simulink model "cf_main_7_2"  (R2022a)
settings: Solver=FixedStepAuto  StartTime=0.0  StopTime=simTime  FixedStep=sample_time  RelTol=1e-3
model workspace: external: MAT-File (data not in the file)
undefined symbols (not defined in the file or in its folder): Angular, g, l0, l1, Linear, mass_total, poly_traj, pos_Kd, pos_Ki, pos_Kp, pos_Kvel, pos_N, pos_sat, Pose, Position, posx_Kd, posx_Ki, posx_Kp, posy_Kd, posy_Ki, posy_Kp, posz_Kd, posz_Ki, posz_Kp, publish_rate, quat2rotm, simTime
libraries: robotlib x11, slpidlib x4, simulink_extras x3, simulink x1, vrlib x1
settings Model: Creator=david  LastModifiedBy=dtu31390
settings SolverCC: AlgebraicLoopSolver=TrustRegion
settings DataIOCC: LimitDataPoints=on  MaxDataPoints=10000
settings OptimizationCC: EnhancedBackFolding=on  PassReuseOutputArgsThreshold=0  ZeroExternalMemoryAtStartup=off  ZeroInternalMemoryAtStartup=off  MaxStackSize=64  OptimizeBlockOrder=speed  DifferentSizesBufferReuse=on
settings DebuggingCC: ParameterTunabilityLossMsg=error  UnconnectedInputMsg=warning  UnconnectedOutputMsg=warning  UnconnectedLineMsg=warning  AllowSymbolicDim=off  SFUnexpectedBacktrackingDiag=warning  SFNoUnconditionalDefaultTransitionDiag=warning  SFExecutionAtInitializationDiag=none  SFMachineParentedDataDiag=warning  UnderSpecifiedDimensionMsg=warning  ArithmeticOperatorsInVariantConditions=warning
settings HardwareCC: ProdBitPerPointer=32  ProdBitPerSizeT=32  ProdBitPerPtrDiffT=32  ProdLargestAtomicFloat=None  ProdIntDivRoundTo=Undefined  ProdEndianess=Unspecified  ProdWordSize=32  ProdHWDeviceType=Generic->Unspecified (assume 32-bit Generic)  UseEmbeddedCoderFeatures=off
settings SFSimCC: SimUseLocalCustomCode=off  MATLABDynamicMemAlloc=off  CustomCodeUndefinedFunction=UseInterfaceOnly  SimTargetLang=C++
settings RTWCC: SystemTargetFile=ert.tlc  HardwareBoard=Robot Operating System (ROS)  TLCOptions="-aInlineSetEventsForThisBaseRateFcn=TLC_FALSE -aSuppressMultiTaskScheduler=TLC_FALSE  -aRateBasedStepFcn=0"  TemplateMakefile=ert_default_tmf  RTWUseLocalCustomCode=off  Toolchain=Catkin  TargetLang=C++  DLArmComputeVersion=19.05
settings CodeAppCC: ForceParamTrailComments=on  OperatorAnnotations=on
settings ERTTargetCC: ERTCustomFileBanners=off  CodeInterfacePackaging=C++ class  SupportContinuousTime=on  SupportNonInlinedSFcns=on  RemoveResetFunc=off  ModelStepFunctionPrototypeControlCompliant=off  RootIOFormat=Structure reference
settings ConfigComp: CovMetricSettings=dw  CovSaveCumulativeToWorkspaceVar=on  CovSaveSingleToWorkspaceVar=on  CovExternalEMLEnable=off  CovSFcnEnable=off
settings SimscapeCC: SimscapeLogType=all  SimscapeLogSimulationStatistics=on  SimscapeLogDataHistory=10000
settings ExplorerConfigSet: InternalSimMechanicsExplorerSettings="<ExplorerConfiguration><canonicalview>default</canonicalview><AnimationSetting><BasePlaybackSpeed>1.0</BasePlaybackSpeed><PlaybackSpeedFactor>1.0</PlaybackSpeedFactor></AnimationSetting><TilePanel><TileInfo><Tiles Columns=\"1\" Count=\"1\" Rows=\"1\"><Column Weight=\"1\"/><Row Weight=\"1\"/><Tile Height=\"1\" Width=\"1\" X=\"0\" Y=\"0\"/></Tiles></TileInfo><SceneInfo><SceneViewer><BGColor><R>0.400000005960464478</R><G>0.400000005960464478</G><B>0.400000005960464478</B></BGColor><Camera><DoPerspective>off</DoPerspective><Position><X>7.41918867546502359</X><Y>0.562842449888731333</Y><Z>8.36768126399918444</Z></Position><Center><X>4.24878770726833288</X><Y>4.27540210027623324</Y><Z>0.996100590645515815</Z></Center><Up><X>-0.578313069199200891</X><Y>0.601173295476169489</Y><Z>0.551493121262380703</Z></Up><ViewLimDist>1</ViewLimDist><YLim>5.48746925830841104</YLim><XLim>8.41878250057976274</XLim></Camera></SceneViewer></SceneInfo></TilePanel><MechEditorPanel><Cameras/><GfxPanelCameraMap/><VideoCreator><PlaybackSpeedRatio>1.0</PlaybackSpeedRatio><FrameRate>30</FrameRate><VideoFormat>Motion JPEG AVI</VideoFormat><FrameSize>auto</FrameSize></VideoCreator></MechEditorPanel></ExplorerConfiguration>"

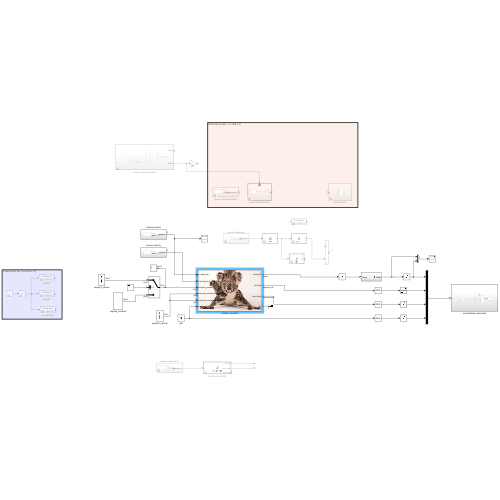
[thumbnail: Simulink's stored preview of the top-level diagram]
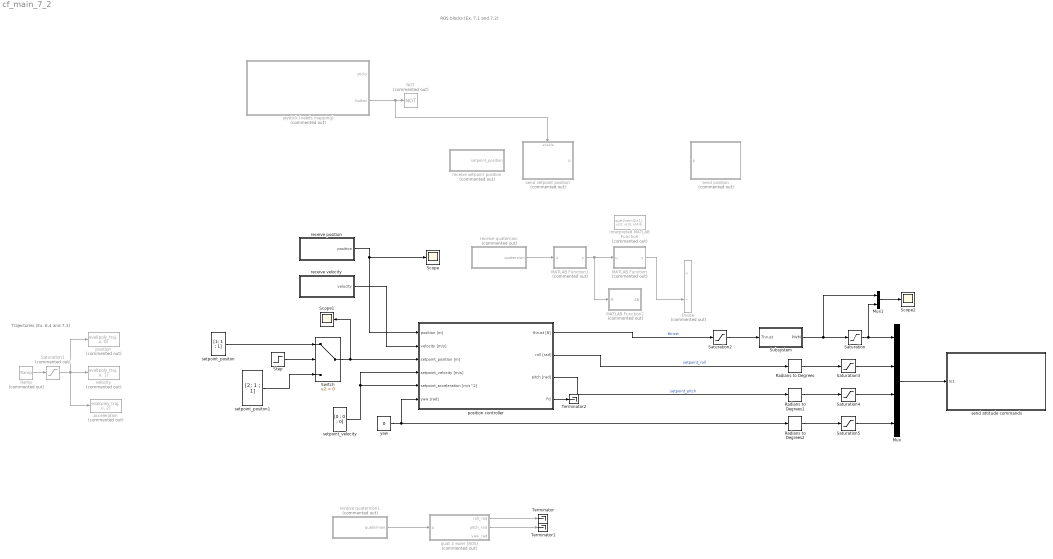
== system cf_main_7_2 ==
  note: Trajectories (Ex. 6.4 and 7.3)
  note: ROS blocks (Ex. 7.1 and 7.2)
  Divide : Product  Commented=on  Inputs=*/
  Interpreted MATLAB Function : MATLABFcn  Commented=on  MATLABFcn=quat2rotm([u(1), u(2), u(3), u(4)])  Output1D=off
  MATLAB Function : MATLAB Function  Commented=on  TreatAsAtomicUnit=on
  MATLAB Function1 : MATLAB Function  Commented=on  TreatAsAtomicUnit=on
  MATLAB Function2 : MATLAB Function  Commented=on  TreatAsAtomicUnit=on
  Mux : Mux
  Mux1 : Mux  Inputs=2
  NOT : Logic  Commented=on  Operator=NOT  IconShape=distinctive  AllPortsSameDT=off  OutDataTypeStr=boolean
  Radians to Degrees : simulink_extras/Transformations/Radians to Degrees
  Radians to Degrees1 : simulink_extras/Transformations/Radians to Degrees
  Radians to Degrees2 : simulink_extras/Transformations/Radians to Degrees
  Ramp : simulink/Sources/Ramp  Commented=on  slope=1  start=0  InitialOutput=0
  Saturation : Saturate  UpperLimit=60000  LowerLimit=0
  Saturation1 : Saturate  Commented=on  UpperLimit=knots(end)  LowerLimit=0
  Saturation2 : Saturate  UpperLimit=0.43  LowerLimit=0
  Saturation3 : Saturate  UpperLimit=5  LowerLimit=-5
  Saturation4 : Saturate  UpperLimit=5  LowerLimit=-5
  Saturation5 : Saturate  UpperLimit=10  LowerLimit=-10
  Scope : Scope
  Scope1 : Scope
  Scope2 : Scope
  Step : Step  Time=simTime-6  Before=1  After=-1  SampleTime=0
  Subsystem : Subsystem
  Switch : Switch  Criteria=u2 > Threshold  SaturateOnIntegerOverflow=off  InputSameDT=off
  Terminator : Terminator
  Terminator1 : Terminator
  Terminator2 : Terminator
  acceleration : MATLABFcn  Commented=on  MATLABFcn=eval(poly_traj, u, 2)  OutputDimensions=[3 1]  Output1D=off
  joystick (needs mapping) : Subsystem  Commented=on
  position : MATLABFcn  Commented=on  MATLABFcn=eval(poly_traj, u, 0)  OutputDimensions=[3 1]  Output1D=off
  position controller : Subsystem
      mask Display: image('$imagefile'); % Use "Edit Image" on toolstrip to change.
  quat 2 euler (ROS) : MATLAB Function  Commented=on  TreatAsAtomicUnit=on
  receive position : Subsystem
  receive quaternion : Subsystem  Commented=on
  receive quaternion1 : Subsystem  Commented=on
  receive setpoint position : Subsystem  Commented=on
  receive velocity : Subsystem
  send attitude commands : Subsystem
  send position : Subsystem  Commented=on
  send setpoint position : Subsystem  Commented=on
  setpoint_positon : Constant  Value=[1; 1 ; 1]  VectorParams1D=off
  setpoint_positon1 : Constant  Value=[2; 1 ; 1]  VectorParams1D=off
  setpoint_velocity : Constant  Value=[0 ; 0 ; 0]  VectorParams1D=off
  velocity : MATLABFcn  Commented=on  MATLABFcn=eval(poly_traj, u, 1)  OutputDimensions=[3 1]  Output1D=off
  yaw : Constant  Value=0
  wires:
  Saturation1/1 -> acceleration/1, position/1, velocity/1
  Ramp/1 -> Saturation1/1
  setpoint_velocity/1 -> position controller/5(setpoint_acceleration [m/s^2]), position controller/4(setpoint_velocity [m/s])
  joystick (needs mapping)/2(button) -> NOT/1, send setpoint position/Enable
  Switch/1 -> position controller/3(setpoint_position [m]), Scope1/1
  Step/1 -> Switch/2
  setpoint_positon/1 -> Switch/1
  setpoint_positon1/1 -> Switch/3
  receive velocity/1(velocity) -> position controller/2(velocity [m/s])
  MATLAB Function/1(y) -> Divide/2
  Mux/1 -> send attitude commands/1(In1)
  position controller/2(roll [rad]) -> Radians to Degrees/1  "setpoint_roll"
  position controller/3(pitch [rad]) -> Radians to Degrees1/1  "setpoint_pitch"
  Subsystem/1(PWM) -> Mux1/1, Saturation/1
  receive quaternion1/1(quaternion) -> quat 2 euler (ROS)/1(q)
  quat 2 euler (ROS)/1(roll_rad) -> Terminator/1
  quat 2 euler (ROS)/2(pitch_rad) -> Terminator1/1
  yaw/1 -> Radians to Degrees2/1, position controller/6(yaw [rad])
  receive position/1(position) -> position controller/1(position [m]), Scope/1
  Saturation/1 -> Mux1/2, Mux/1
  Mux1/1 -> Scope2/1
  Radians to Degrees1/1 -> Saturation4/1
  Saturation4/1 -> Mux/3
  Radians to Degrees/1 -> Saturation3/1
  Saturation3/1 -> Mux/2
  Radians to Degrees2/1 -> Saturation5/1
  Saturation5/1 -> Mux/4
  Saturation2/1 -> Subsystem/1(Thrust)
  receive quaternion/1(quaternion) -> MATLAB Function1/1(u)
  MATLAB Function1/1(y) -> MATLAB Function2/1(R), MATLAB Function/1(u)
  position controller/4(Fd) -> Terminator2/1
  position controller/1(thrust [N]) -> Saturation2/1  "thrust"

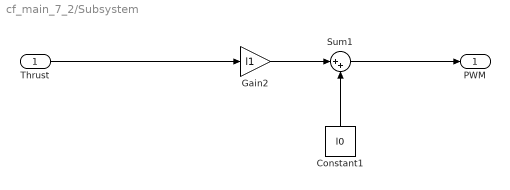
== system cf_main_7_2/Subsystem ==
  Thrust : Inport
  Constant1 : Constant  Value=l0
  Gain2 : Gain  Gain=l1
  Sum1 : Sum  Inputs=|++
  PWM : Outport
  wires:
  Thrust/1 -> Gain2/1
  Sum1/1 -> PWM/1
  Constant1/1 -> Sum1/2
  Gain2/1 -> Sum1/1

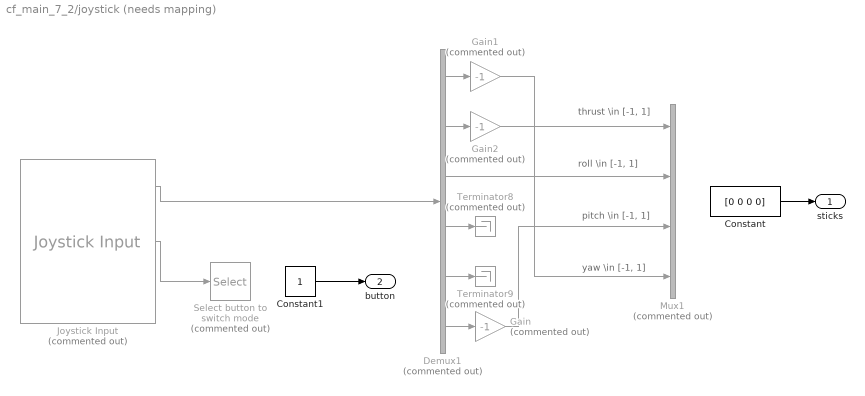
== system cf_main_7_2/joystick (needs mapping) ==
  note: thrust \in [-1, 1]
  note: roll \in [-1, 1]
  note: pitch \in [-1, 1]
  note: yaw \in [-1, 1]
  Constant : Constant  Value=[0 0 0 0]
  Constant1 : Constant
  Demux1 : Demux  Commented=on  Outputs=6
  Gain : Gain  Commented=on  Gain=-1
  Gain1 : Gain  Commented=on  Gain=-1
  Gain2 : Gain  Commented=on  Gain=-1
  Joystick Input : vrlib/Joystick Input  Commented=on  joyid=1  adjustports=on  forcefeed=off
  Mux1 : Mux  Commented=on
  Select button to switch mode : Selector  Commented=on  InputPortWidth=15  IndexOptions=Index vector (dialog)  Indices=8  OutputSizes=1
  Terminator8 : Terminator  Commented=on
  Terminator9 : Terminator  Commented=on
  sticks : Outport
  button : Outport  Port=2
  wires:
  Gain1/1 -> Mux1/4
  Joystick Input/1 -> Demux1/1
  Gain2/1 -> Mux1/1
  Demux1/1 -> Gain1/1
  Joystick Input/2 -> Select button to switch mode/1
  Demux1/6 -> Gain/1
  Demux1/5 -> Terminator9/1
  Demux1/3 -> Mux1/2
  Demux1/2 -> Gain2/1
  Demux1/4 -> Terminator8/1
  Gain/1 -> Mux1/3
  Constant/1 -> sticks/1
  Constant1/1 -> button/1

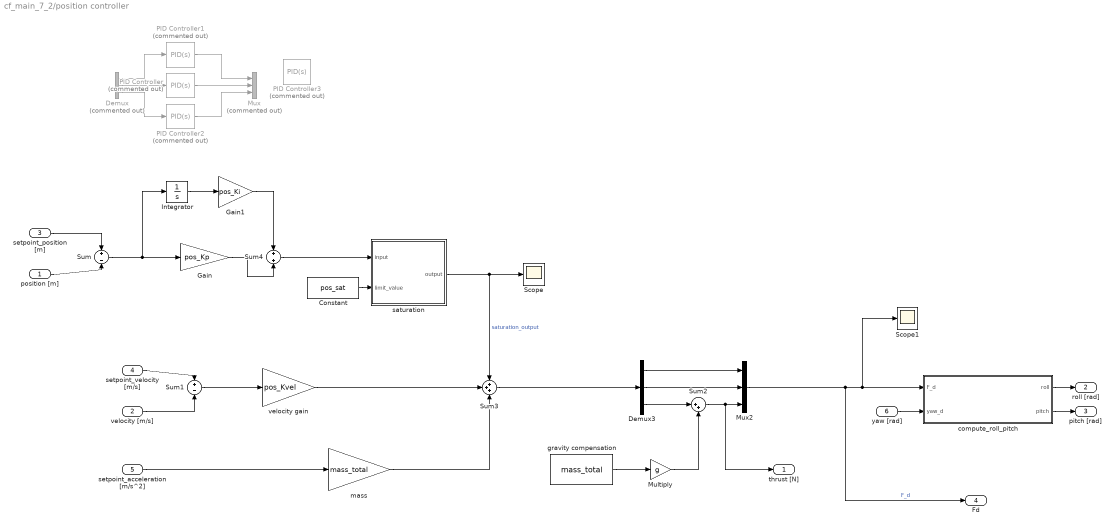
== system cf_main_7_2/position controller ==
  position [m] : Inport
  velocity [m/s] : Inport  Port=2
  setpoint_position [m] : Inport  Port=3
  setpoint_velocity [m/s] : Inport  Port=4
  setpoint_acceleration [m/s^2] : Inport  Port=5
  yaw [rad] : Inport  Port=6
  Constant : Constant  Value=pos_sat
  Demux : Demux  Commented=on  Outputs=3
  Demux3 : Demux  Outputs=3
  Gain : Gain  Gain=pos_Kp
  Gain1 : Gain  Gain=pos_Ki
  Integrator : Integrator
  Multiply : Gain  Gain=g
  Mux : Mux  Commented=on  Inputs=3
  Mux2 : Mux  Inputs=3
  PID Controller : slpidlib/PID Controller  Commented=on  Controller=PID  Form=Parallel  TimeDomain=Continuous-time  UseExternalTs=off  SampleTime=-1  IntegratorMethod=Forward Euler  FilterMethod=Forward Euler  ControllerParametersSource=internal  P=posy_Kp  I=posy_Ki  UseKiTs=off  D=posy_Kd  N=pos_N  UseFilter=on  TunerSelectOption=Transfer Function Based (PID Tuner App)  InitialConditionSource=internal  InitialConditionForIntegrator=0  InitialConditionForFilter=0  DifferentiatorICPrevScaledInput=0  ExternalReset=none  TrackingMode=off  Kt=1  LimitOutput=off  SatLimitsSource=internal  UpperSaturationLimit=inf  LowerSaturationLimit=-inf  LinearizeAsGain=on  AntiWindupMode=none  Kb=1  POutMin=[]  POutMax=[]  IOutMin=[]  IOutMax=[]  DOutMin=[]  DOutMax=[]  NOutMin=[]  NOutMax=[]  SumOutMin=[]  SumOutMax=[]  SaturationOutMin=[]  SaturationOutMax=[]  PParamMin=[]  PParamMax=[]  IParamMin=[]  IParamMax=[]  DParamMin=[]  DParamMax=[]  NParamMin=[]  NParamMax=[]  KbParamMin=[]  KbParamMax=[]  KtParamMin=[]  KtParamMax=[]  KbOutMin=[]  KbOutMax=[]  KtOutMin=[]  KtOutMax=[]  IntegratorOutMin=[]  IntegratorOutMax=[]  FilterOutMin=[]  FilterOutMax=[]  SumI1OutMin=[]  SumI1OutMax=[]  SumI2OutMin=[]  SumI2OutMax=[]  SumI3OutMin=[]  SumI3OutMax=[]  SumI4OutMin=[]  SumI4OutMax=[]  SumDOutMin=[]  SumDOutMax=[]  DifferentiatorOutMin=[]  DifferentiatorOutMax=[]  FilterDiffOutCoefMin=[]  FilterDiffOutCoefMax=[]  ReciprocalOutMin=[]  ReciprocalOutMax=[]  SumDenOutMin=[]  SumDenOutMax=[]  SumNumOutMin=[]  SumNumOutMax=[]  DivideOutMin=[]  DivideOutMax=[]  UdiffTsProdOutMin=[]  UdiffTsProdOutMax=[]  NTsProdOutMin=[]  NTsProdOutMax=[]  UintegralTsProdOutMin=[]  UintegralTsProdOutMax=[]  UngainTsProdOutMin=[]  UngainTsProdOutMax=[]  IntegratorContinuousStateAttributes=''  IntegratorStateMustResolveToSignalObject=off  IntegratorRTWStateStorageClass=Auto  FilterContinuousStateAttributes=''  FilterStateMustResolveToSignalObject=off  FilterRTWStateStorageClass=Auto  ParallelPVariant=InternalParameters  IdealPVariant=Disabled  IVariant=InternalParameters  DVariant=InternalParameters  IntegratorVariant=Continuous  SatVariant=Disabled  AWVariant=Passthrough  PCopyVariant=Disabled  TRVariant=Disabled  FdbkBlocksVariant=Forward  IdealPFdbkVariant=Disabled  SatFdbkVariant=Disabled  DerivativeFilterVariant=ContFilter  NVariant=InternalParameters  NCopyVariant=Disabled  FilterICVariant=InternalICsFilter  IntegratorICVariant=InternalICs  ExternalResetVariant=Disabled  TRSumVariant=Passthrough  SumFdbkVariant=Disabled  SumVariant=Sum_PID  TsampFilterVariant=InternalTs  TsampNgainVariant=Passthrough  TsampIntegralVariant=Passthrough  ExternalSaturationOutDataTypeStr=Inherit: Same as second input  aMode=0
  PID Controller1 : slpidlib/PID Controller  Commented=on  Controller=PID  Form=Parallel  TimeDomain=Continuous-time  UseExternalTs=off  SampleTime=-1  IntegratorMethod=Forward Euler  FilterMethod=Forward Euler  ControllerParametersSource=internal  P=posx_Kp  I=posx_Ki  UseKiTs=off  D=posx_Kd  N=pos_N  UseFilter=on  TunerSelectOption=Transfer Function Based (PID Tuner App)  InitialConditionSource=internal  InitialConditionForIntegrator=0  InitialConditionForFilter=0  DifferentiatorICPrevScaledInput=0  ExternalReset=none  TrackingMode=off  Kt=1  LimitOutput=off  SatLimitsSource=internal  UpperSaturationLimit=inf  LowerSaturationLimit=-inf  LinearizeAsGain=on  AntiWindupMode=none  Kb=1  POutMin=[]  POutMax=[]  IOutMin=[]  IOutMax=[]  DOutMin=[]  DOutMax=[]  NOutMin=[]  NOutMax=[]  SumOutMin=[]  SumOutMax=[]  SaturationOutMin=[]  SaturationOutMax=[]  PParamMin=[]  PParamMax=[]  IParamMin=[]  IParamMax=[]  DParamMin=[]  DParamMax=[]  NParamMin=[]  NParamMax=[]  KbParamMin=[]  KbParamMax=[]  KtParamMin=[]  KtParamMax=[]  KbOutMin=[]  KbOutMax=[]  KtOutMin=[]  KtOutMax=[]  IntegratorOutMin=[]  IntegratorOutMax=[]  FilterOutMin=[]  FilterOutMax=[]  SumI1OutMin=[]  SumI1OutMax=[]  SumI2OutMin=[]  SumI2OutMax=[]  SumI3OutMin=[]  SumI3OutMax=[]  SumI4OutMin=[]  SumI4OutMax=[]  SumDOutMin=[]  SumDOutMax=[]  DifferentiatorOutMin=[]  DifferentiatorOutMax=[]  FilterDiffOutCoefMin=[]  FilterDiffOutCoefMax=[]  ReciprocalOutMin=[]  ReciprocalOutMax=[]  SumDenOutMin=[]  SumDenOutMax=[]  SumNumOutMin=[]  SumNumOutMax=[]  DivideOutMin=[]  DivideOutMax=[]  UdiffTsProdOutMin=[]  UdiffTsProdOutMax=[]  NTsProdOutMin=[]  NTsProdOutMax=[]  UintegralTsProdOutMin=[]  UintegralTsProdOutMax=[]  UngainTsProdOutMin=[]  UngainTsProdOutMax=[]  IntegratorContinuousStateAttributes=''  IntegratorStateMustResolveToSignalObject=off  IntegratorRTWStateStorageClass=Auto  FilterContinuousStateAttributes=''  FilterStateMustResolveToSignalObject=off  FilterRTWStateStorageClass=Auto  ParallelPVariant=InternalParameters  IdealPVariant=Disabled  IVariant=InternalParameters  DVariant=InternalParameters  IntegratorVariant=Continuous  SatVariant=Disabled  AWVariant=Passthrough  PCopyVariant=Disabled  TRVariant=Disabled  FdbkBlocksVariant=Forward  IdealPFdbkVariant=Disabled  SatFdbkVariant=Disabled  DerivativeFilterVariant=ContFilter  NVariant=InternalParameters  NCopyVariant=Disabled  FilterICVariant=InternalICsFilter  IntegratorICVariant=InternalICs  ExternalResetVariant=Disabled  TRSumVariant=Passthrough  SumFdbkVariant=Disabled  SumVariant=Sum_PID  TsampFilterVariant=InternalTs  TsampNgainVariant=Passthrough  TsampIntegralVariant=Passthrough  ExternalSaturationOutDataTypeStr=Inherit: Same as second input  aMode=0
  PID Controller2 : slpidlib/PID Controller  Commented=on  Controller=PID  Form=Parallel  TimeDomain=Continuous-time  UseExternalTs=off  SampleTime=-1  IntegratorMethod=Forward Euler  FilterMethod=Forward Euler  ControllerParametersSource=internal  P=posz_Kp  I=posz_Ki  UseKiTs=off  D=posz_Kd  N=pos_N  UseFilter=on  TunerSelectOption=Transfer Function Based (PID Tuner App)  InitialConditionSource=internal  InitialConditionForIntegrator=0  InitialConditionForFilter=0  DifferentiatorICPrevScaledInput=0  ExternalReset=none  TrackingMode=off  Kt=1  LimitOutput=off  SatLimitsSource=internal  UpperSaturationLimit=inf  LowerSaturationLimit=-inf  LinearizeAsGain=on  AntiWindupMode=none  Kb=1  POutMin=[]  POutMax=[]  IOutMin=[]  IOutMax=[]  DOutMin=[]  DOutMax=[]  NOutMin=[]  NOutMax=[]  SumOutMin=[]  SumOutMax=[]  SaturationOutMin=[]  SaturationOutMax=[]  PParamMin=[]  PParamMax=[]  IParamMin=[]  IParamMax=[]  DParamMin=[]  DParamMax=[]  NParamMin=[]  NParamMax=[]  KbParamMin=[]  KbParamMax=[]  KtParamMin=[]  KtParamMax=[]  KbOutMin=[]  KbOutMax=[]  KtOutMin=[]  KtOutMax=[]  IntegratorOutMin=[]  IntegratorOutMax=[]  FilterOutMin=[]  FilterOutMax=[]  SumI1OutMin=[]  SumI1OutMax=[]  SumI2OutMin=[]  SumI2OutMax=[]  SumI3OutMin=[]  SumI3OutMax=[]  SumI4OutMin=[]  SumI4OutMax=[]  SumDOutMin=[]  SumDOutMax=[]  DifferentiatorOutMin=[]  DifferentiatorOutMax=[]  FilterDiffOutCoefMin=[]  FilterDiffOutCoefMax=[]  ReciprocalOutMin=[]  ReciprocalOutMax=[]  SumDenOutMin=[]  SumDenOutMax=[]  SumNumOutMin=[]  SumNumOutMax=[]  DivideOutMin=[]  DivideOutMax=[]  UdiffTsProdOutMin=[]  UdiffTsProdOutMax=[]  NTsProdOutMin=[]  NTsProdOutMax=[]  UintegralTsProdOutMin=[]  UintegralTsProdOutMax=[]  UngainTsProdOutMin=[]  UngainTsProdOutMax=[]  IntegratorContinuousStateAttributes=''  IntegratorStateMustResolveToSignalObject=off  IntegratorRTWStateStorageClass=Auto  FilterContinuousStateAttributes=''  FilterStateMustResolveToSignalObject=off  FilterRTWStateStorageClass=Auto  ParallelPVariant=InternalParameters  IdealPVariant=Disabled  IVariant=InternalParameters  DVariant=InternalParameters  IntegratorVariant=Continuous  SatVariant=Disabled  AWVariant=Passthrough  PCopyVariant=Disabled  TRVariant=Disabled  FdbkBlocksVariant=Forward  IdealPFdbkVariant=Disabled  SatFdbkVariant=Disabled  DerivativeFilterVariant=ContFilter  NVariant=InternalParameters  NCopyVariant=Disabled  FilterICVariant=InternalICsFilter  IntegratorICVariant=InternalICs  ExternalResetVariant=Disabled  TRSumVariant=Passthrough  SumFdbkVariant=Disabled  SumVariant=Sum_PID  TsampFilterVariant=InternalTs  TsampNgainVariant=Passthrough  TsampIntegralVariant=Passthrough  ExternalSaturationOutDataTypeStr=Inherit: Same as second input  aMode=0
  PID Controller3 : slpidlib/PID Controller  Commented=on  Controller=PID  Form=Parallel  TimeDomain=Continuous-time  UseExternalTs=off  SampleTime=-1  IntegratorMethod=Forward Euler  FilterMethod=Forward Euler  ControllerParametersSource=internal  P=pos_Kp  I=pos_Ki  UseKiTs=off  D=pos_Kd  N=pos_N  UseFilter=on  TunerSelectOption=Transfer Function Based (PID Tuner App)  InitialConditionSource=internal  InitialConditionForIntegrator=0  InitialConditionForFilter=0  DifferentiatorICPrevScaledInput=0  ExternalReset=none  TrackingMode=off  Kt=1  LimitOutput=off  SatLimitsSource=internal  UpperSaturationLimit=inf  LowerSaturationLimit=-inf  LinearizeAsGain=on  AntiWindupMode=none  Kb=1  POutMin=[]  POutMax=[]  IOutMin=[]  IOutMax=[]  DOutMin=[]  DOutMax=[]  NOutMin=[]  NOutMax=[]  SumOutMin=[]  SumOutMax=[]  SaturationOutMin=[]  SaturationOutMax=[]  PParamMin=[]  PParamMax=[]  IParamMin=[]  IParamMax=[]  DParamMin=[]  DParamMax=[]  NParamMin=[]  NParamMax=[]  KbParamMin=[]  KbParamMax=[]  KtParamMin=[]  KtParamMax=[]  KbOutMin=[]  KbOutMax=[]  KtOutMin=[]  KtOutMax=[]  IntegratorOutMin=[]  IntegratorOutMax=[]  FilterOutMin=[]  FilterOutMax=[]  SumI1OutMin=[]  SumI1OutMax=[]  SumI2OutMin=[]  SumI2OutMax=[]  SumI3OutMin=[]  SumI3OutMax=[]  SumI4OutMin=[]  SumI4OutMax=[]  SumDOutMin=[]  SumDOutMax=[]  DifferentiatorOutMin=[]  DifferentiatorOutMax=[]  FilterDiffOutCoefMin=[]  FilterDiffOutCoefMax=[]  ReciprocalOutMin=[]  ReciprocalOutMax=[]  SumDenOutMin=[]  SumDenOutMax=[]  SumNumOutMin=[]  SumNumOutMax=[]  DivideOutMin=[]  DivideOutMax=[]  UdiffTsProdOutMin=[]  UdiffTsProdOutMax=[]  NTsProdOutMin=[]  NTsProdOutMax=[]  UintegralTsProdOutMin=[]  UintegralTsProdOutMax=[]  UngainTsProdOutMin=[]  UngainTsProdOutMax=[]  IntegratorContinuousStateAttributes=''  IntegratorStateMustResolveToSignalObject=off  IntegratorRTWStateStorageClass=Auto  FilterContinuousStateAttributes=''  FilterStateMustResolveToSignalObject=off  FilterRTWStateStorageClass=Auto  ParallelPVariant=InternalParameters  IdealPVariant=Disabled  IVariant=InternalParameters  DVariant=InternalParameters  IntegratorVariant=Continuous  SatVariant=Disabled  AWVariant=Passthrough  PCopyVariant=Disabled  TRVariant=Disabled  FdbkBlocksVariant=Forward  IdealPFdbkVariant=Disabled  SatFdbkVariant=Disabled  DerivativeFilterVariant=ContFilter  NVariant=InternalParameters  NCopyVariant=Disabled  FilterICVariant=InternalICsFilter  IntegratorICVariant=InternalICs  ExternalResetVariant=Disabled  TRSumVariant=Passthrough  SumFdbkVariant=Disabled  SumVariant=Sum_PID  TsampFilterVariant=InternalTs  TsampNgainVariant=Passthrough  TsampIntegralVariant=Passthrough  ExternalSaturationOutDataTypeStr=Inherit: Same as second input  aMode=0
  Scope : Scope
  Scope1 : Scope
  Sum : Sum  Inputs=+|-
  Sum1 : Sum  Inputs=+|-
  Sum2 : Sum  Inputs=|++
  Sum3 : Sum  Inputs=+++
  Sum4 : Sum
  compute_roll_pitch : MATLAB Function  TreatAsAtomicUnit=on
  gravity compensation : Constant  Value=mass_total  VectorParams1D=off
  mass : Gain  Gain=mass_total
  saturation : Subsystem
  velocity gain : Gain  Gain=pos_Kvel
  thrust [N] : Outport
  roll [rad] : Outport  Port=2
  pitch [rad] : Outport  Port=3
  Fd : Outport  Port=4
  wires:
  gravity compensation/1 -> Multiply/1
  velocity [m/s]/1 -> Sum1/2
  Demux3/3 -> Sum2/1
  Constant/1 -> saturation/2(limit_value)
  Sum2/1 -> thrust [N]/1, Mux2/3
  Sum1/1 -> velocity gain/1
  velocity gain/1 -> Sum3/2
  Demux3/1 -> Mux2/1
  Mux2/1 -> Fd/1, Scope1/1, compute_roll_pitch/1(F_d)  "F_d"
  Demux3/2 -> Mux2/2
  compute_roll_pitch/1(roll) -> roll [rad]/1
  Multiply/1 -> Sum2/2
  setpoint_position [m]/1 -> Sum/1
  compute_roll_pitch/2(pitch) -> pitch [rad]/1
  position [m]/1 -> Sum/2
  yaw [rad]/1 -> compute_roll_pitch/2(yaw_d)
  setpoint_velocity [m/s]/1 -> Sum1/1
  Demux/1 -> PID Controller1/1
  Demux/2 -> PID Controller/1
  PID Controller/1 -> Mux/2
  Demux/3 -> PID Controller2/1
  PID Controller2/1 -> Mux/3
  PID Controller1/1 -> Mux/1
  setpoint_acceleration [m/s^2]/1 -> mass/1
  Sum3/1 -> Demux3/1
  mass/1 -> Sum3/3
  saturation/1(output) -> Sum3/1, Scope/1  "saturation_output"
  Gain/1 -> Sum4/2
  Integrator/1 -> Gain1/1
  Gain1/1 -> Sum4/1
  Sum4/1 -> saturation/1(input)
  Sum/1 -> Integrator/1, Gain/1

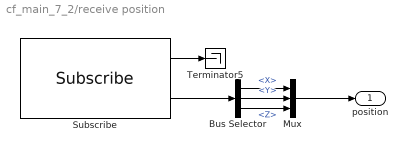
== system cf_main_7_2/receive position ==
  Bus Selector : BusSelector  OutputSignals=Pose.Position.X,Pose.Position.Y,Pose.Position.Z
  Mux : Mux  Inputs=3
  Subscribe : robotlib/Subscribe  topicSource=Select from ROS network  topic=/crazyflie/pose  messageType=geometry_msgs/PoseStamped  SampleTime=-1  legacyBusStruct=off  messageQueueLength=1
  Terminator5 : Terminator
  position : Outport
  wires:
  Subscribe/2 -> Bus Selector/1
  Mux/1 -> position/1
  Bus Selector/3 -> Mux/3  "<Z>"
  Bus Selector/1 -> Mux/1  "<X>"
  Bus Selector/2 -> Mux/2  "<Y>"
  Subscribe/1 -> Terminator5/1

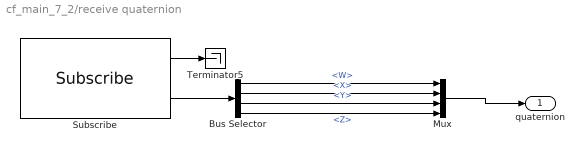
== system cf_main_7_2/receive quaternion ==
  Bus Selector : BusSelector  OutputSignals=Pose.Orientation.W,Pose.Orientation.X,Pose.Orientation.Y,Pose.Orientation.Z
  Mux : Mux
  Subscribe : robotlib/Subscribe  topicSource=Select from ROS network  topic=/crazyflie/pose  messageType=geometry_msgs/PoseStamped  SampleTime=-1  legacyBusStruct=off  messageQueueLength=1
  Terminator5 : Terminator
  quaternion : Outport
  wires:
  Subscribe/2 -> Bus Selector/1
  Mux/1 -> quaternion/1
  Bus Selector/3 -> Mux/3  "<Y>"
  Bus Selector/1 -> Mux/1  "<W>"
  Bus Selector/2 -> Mux/2  "<X>"
  Subscribe/1 -> Terminator5/1
  Bus Selector/4 -> Mux/4  "<Z>"

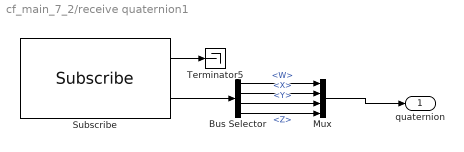
== system cf_main_7_2/receive quaternion1 ==
  Bus Selector : BusSelector  OutputSignals=Pose.Orientation.W,Pose.Orientation.X,Pose.Orientation.Y,Pose.Orientation.Z
  Mux : Mux
  Subscribe : robotlib/Subscribe  topicSource=Select from ROS network  topic=/crazyflie/pose  messageType=geometry_msgs/PoseStamped  SampleTime=-1  legacyBusStruct=off  messageQueueLength=1
  Terminator5 : Terminator
  quaternion : Outport
  wires:
  Subscribe/2 -> Bus Selector/1
  Mux/1 -> quaternion/1
  Bus Selector/3 -> Mux/3  "<Y>"
  Bus Selector/1 -> Mux/1  "<W>"
  Bus Selector/2 -> Mux/2  "<X>"
  Subscribe/1 -> Terminator5/1
  Bus Selector/4 -> Mux/4  "<Z>"

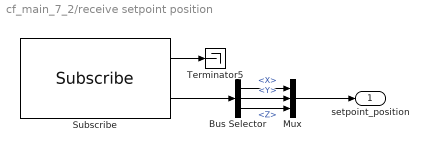
== system cf_main_7_2/receive setpoint position ==
  Bus Selector : BusSelector  OutputSignals=Position.X,Position.Y,Position.Z
  Mux : Mux  Inputs=3
  Subscribe : robotlib/Subscribe  topicSource=Specify your own  topic=/crazyflie/cmd_position  messageType=geometry_msgs/Pose  SampleTime=-1  legacyBusStruct=off  messageQueueLength=1
  Terminator5 : Terminator
  setpoint_position : Outport
  wires:
  Subscribe/2 -> Bus Selector/1
  Mux/1 -> setpoint_position/1
  Bus Selector/3 -> Mux/3  "<Z>"
  Bus Selector/1 -> Mux/1  "<X>"
  Bus Selector/2 -> Mux/2  "<Y>"
  Subscribe/1 -> Terminator5/1

== system cf_main_7_2/receive velocity ==
  Bus Selector : BusSelector  OutputSignals=Twist.Linear.X,Twist.Linear.Y,Twist.Linear.Z
  Mux : Mux  Inputs=3
  Subscribe : robotlib/Subscribe  topicSource=Specify your own  topic=/crazyflie/twist  messageType=geometry_msgs/TwistStamped  SampleTime=-1  legacyBusStruct=off  messageQueueLength=1
  Terminator5 : Terminator
  velocity : Outport
  wires:
  Subscribe/2 -> Bus Selector/1
  Mux/1 -> velocity/1
  Bus Selector/3 -> Mux/3  "<Z>"
  Bus Selector/1 -> Mux/1  "<X>"
  Bus Selector/2 -> Mux/2  "<Y>"
  Subscribe/1 -> Terminator5/1

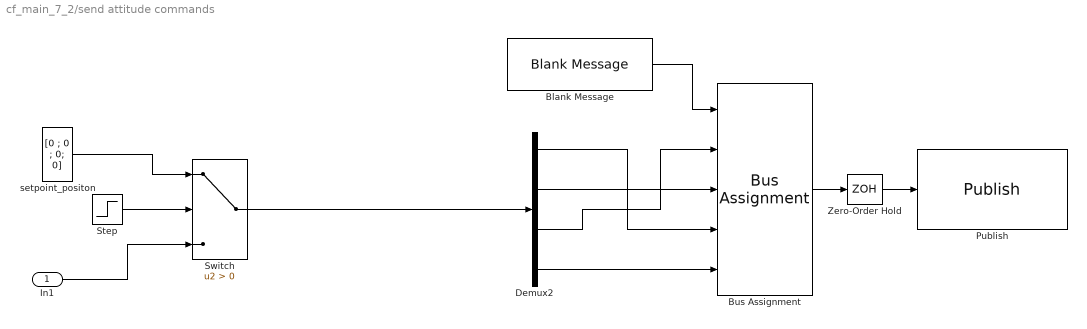
== system cf_main_7_2/send attitude commands ==
  In1 : Inport
  Blank Message : robotlib/Blank Message  messageClass=Message  entityType=geometry_msgs/Twist  messageType=geometry_msgs/Twist  SampleTime=inf  legacyBusStruct=off
  Bus Assignment : BusAssignment  AssignedSignals=Linear.X,Linear.Y,Linear.Z,Angular.Z
  Demux2 : Demux
  Publish : robotlib/Publish  topicSource=Select from ROS network  topic=/crazyflie/cmd_vel  messageType=geometry_msgs/Twist  legacyBusStruct=off  messageQueueLength=1
  Step : Step  Time=2  Before=1  After=-1  SampleTime=0
  Switch : Switch  Criteria=u2 > Threshold  SaturateOnIntegerOverflow=off  InputSameDT=off
  Zero-Order Hold : ZeroOrderHold  SampleTime=1/25
  setpoint_positon : Constant  Value=[0 ; 0 ; 0; 0]  VectorParams1D=off
  wires:
  Zero-Order Hold/1 -> Publish/1
  Blank Message/1 -> Bus Assignment/1
  Bus Assignment/1 -> Zero-Order Hold/1
  Demux2/1 -> Bus Assignment/4
  Demux2/2 -> Bus Assignment/3
  Demux2/3 -> Bus Assignment/2
  Demux2/4 -> Bus Assignment/5
  Step/1 -> Switch/2
  setpoint_positon/1 -> Switch/1
  In1/1 -> Switch/3
  Switch/1 -> Demux2/1

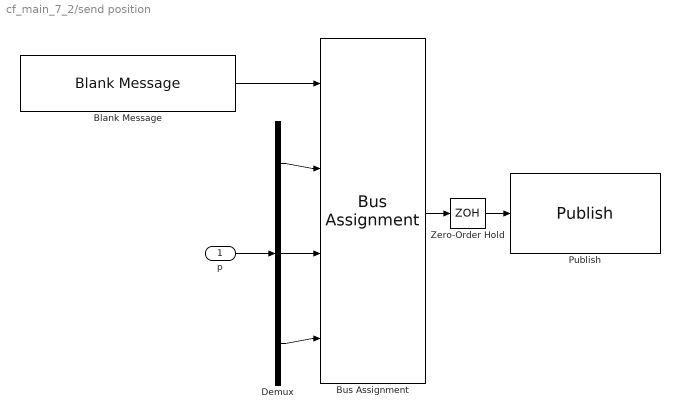
== system cf_main_7_2/send position ==
  p : Inport
  Blank Message : robotlib/Blank Message  messageClass=Message  entityType=geometry_msgs/PoseStamped  messageType=geometry_msgs/PoseStamped  SampleTime=inf  legacyBusStruct=off
  Bus Assignment : BusAssignment  AssignedSignals=Pose.Position.X,Pose.Position.Y,Pose.Position.Z
  Demux : Demux  Outputs=3
  Publish : robotlib/Publish  topicSource=Specify your own  topic=/crazyflie/pose  messageType=geometry_msgs/PoseStamped  legacyBusStruct=off  messageQueueLength=1
  Zero-Order Hold : ZeroOrderHold  SampleTime=publish_rate
  wires:
  Bus Assignment/1 -> Zero-Order Hold/1
  Blank Message/1 -> Bus Assignment/1
  Zero-Order Hold/1 -> Publish/1
  Demux/1 -> Bus Assignment/2
  Demux/2 -> Bus Assignment/3
  Demux/3 -> Bus Assignment/4
  p/1 -> Demux/1

== system cf_main_7_2/send setpoint position ==
  p : Inport
  Enable : EnablePort
  send setpoint position : Subsystem
  wires:
  p/1 -> send setpoint position/1(p)

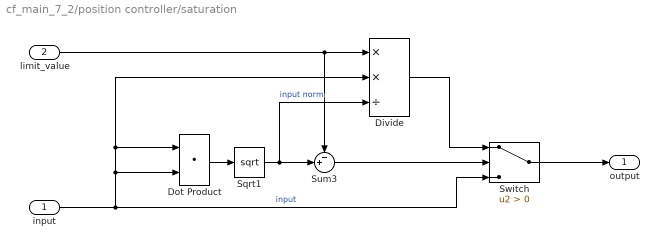
== system cf_main_7_2/position controller/saturation ==
  input : Inport
  limit_value : Inport  Port=2
  Divide : Product  Inputs=**/
  Dot Product : DotProduct  OutDataTypeStr=Inherit: Inherit via internal rule
  Sqrt1 : Sqrt
  Sum3 : Sum  Inputs=-+|
  Switch : Switch  Criteria=u2 > Threshold  SaturateOnIntegerOverflow=off  InputSameDT=off
  output : Outport
  wires:
  Divide/1 -> Switch/1
  limit_value/1 -> Divide/1, Sum3/1
  Dot Product/1 -> Sqrt1/1
  Switch/1 -> output/1
  Sum3/1 -> Switch/2
  input/1 -> Divide/2, Dot Product/1, Dot Product/2, Switch/3  "input"
  Sqrt1/1 -> Divide/3, Sum3/2  "input norm"

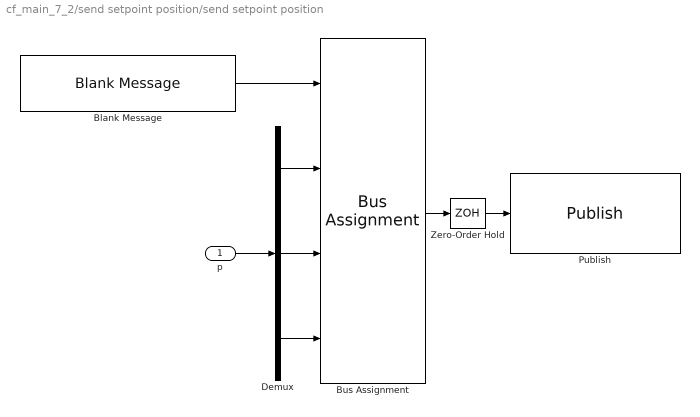
== system cf_main_7_2/send setpoint position/send setpoint position ==
  p : Inport
  Blank Message : robotlib/Blank Message  messageClass=Message  entityType=geometry_msgs/Pose  messageType=geometry_msgs/Pose  SampleTime=inf  legacyBusStruct=off
  Bus Assignment : BusAssignment  AssignedSignals=Position.X,Position.Y,Position.Z
  Demux : Demux  Outputs=3
  Publish : robotlib/Publish  topicSource=Select from ROS network  topic=/crazyflie/cmd_position  messageType=geometry_msgs/Pose  legacyBusStruct=off  messageQueueLength=1
  Zero-Order Hold : ZeroOrderHold  SampleTime=publish_rate
  wires:
  Bus Assignment/1 -> Zero-Order Hold/1
  Blank Message/1 -> Bus Assignment/1
  Zero-Order Hold/1 -> Publish/1
  Demux/1 -> Bus Assignment/2
  Demux/2 -> Bus Assignment/3
  Demux/3 -> Bus Assignment/4
  p/1 -> Demux/1

== matlab function cf_main_7_2/MATLAB Function1 ==
  data: u input; y output
function y = fcn(u)

y = quat2rotm(u');

== matlab function cf_main_7_2/position controller/compute_roll_pitch ==
  data: F_d input; roll output; yaw_d input; pitch output
function [roll, pitch] = compute_roll_pitch(F_d, yaw_d)

yaw_dt = yaw_d + pi/2;
uyt = [cos(yaw_dt); sin(yaw_dt); 0];
uz = F_d/norm(F_d);
ux = cross(uyt, uz);
uy = cross(uz, ux);

attitude = rotm2eul([ux uy uz], 'ZYX');

roll = attitude(3);
pitch = attitude(2);

== matlab function cf_main_7_2/MATLAB Function2 ==
  data: R input; ZB output
function ZB = fcn(R)
ZB = R(:,3);

== matlab function cf_main_7_2/quat 2 euler (ROS) ==
  data: q input size=[1 4]; roll_rad output; pitch_rad output; yaw_rad output
function [roll_rad, pitch_rad, yaw_rad] = euler_ros(q)

attitude = quat2eul(q, 'ZYX');

roll_rad = attitude(3);
pitch_rad = attitude(2);
yaw_rad = attitude(1);

== matlab function cf_main_7_2/MATLAB Function ==
  data: u input; y output
function y = get33(u)

y = u(3,3);
